simulink library "error_sensory_library"  (R2021a)
settings: Solver=VariableStepAuto  StartTime=0.0  StopTime=10.0  RelTol=1e-3
settings Model: Creator=Laura  LastModifiedBy=Laura

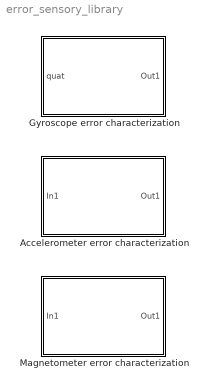
== system error_sensory_library ==
  Accelerometer error characterization : Subsystem
  Gyroscope error characterization : Subsystem
  Magnetometer error characterization : Subsystem

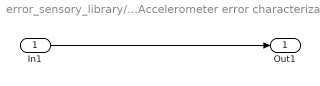
== system error_sensory_library/Accelerometer error characterization ==
  In1 : Inport
  Out1 : Outport
  wires:
  In1/1 -> Out1/1

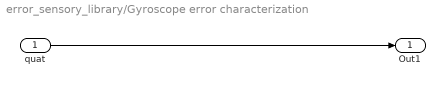
== system error_sensory_library/Gyroscope error characterization ==
  quat : Inport
  Out1 : Outport
  wires:
  quat/1 -> Out1/1

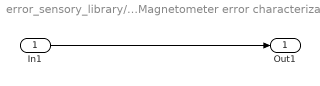
== system error_sensory_library/Magnetometer error characterization ==
  In1 : Inport
  Out1 : Outport
  wires:
  In1/1 -> Out1/1
